simulink model "LHC_18kW_v3"  (R2015a)
settings: Solver=ode15s  StartTime=0.0  StopTime=5e6  MaxStep=1e2  RelTol=1e-3
libraries: simCryogenics_lib x134, nesl_utility x90
(part 2 of 2)

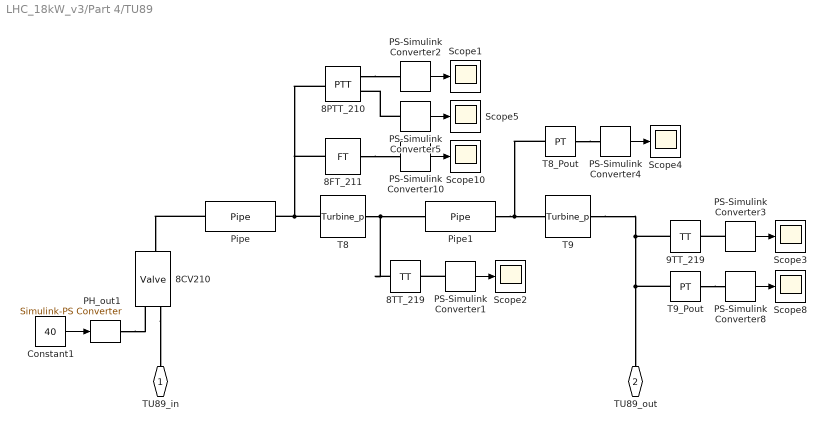
== system LHC_18kW_v3/Part 4/TU89 ==
  8CV210 : simCryogenics_lib/Elements/Valve  CVmax=37  ControlInputMin=0  ControlInputMax=100  Xt=0.65  Rv=50  lin_v=0  lim_v=0  K=2.4e-5 m^1.50000*kg^0.50000/s/bar^0.50000  Cmd_specify=off  Cmd_priority=High  Cmd=0  gamma_specify=off  gamma_priority=High  gamma=0  rho_specify=off  rho_priority=High  rho=0 kg/m^3  Xc_specify=off  Xc_priority=High  Xc=0  X_specify=off  X_priority=High  X=0  Y_specify=off  Y_priority=High  Y=0  CV_specify=off  CV_priority=High  CV=0
  8FT_211 : simCryogenics_lib/Sensors/FT
  8PTT_210 : simCryogenics_lib/Sensors/PTT
  8TT_219 : simCryogenics_lib/Sensors/TT
  9TT_219 : simCryogenics_lib/Sensors/TT
  Constant1 : Constant  Value=40
  PH_out1 : nesl_utility/Simulink-PS Converter  PhysicalDomain=network_engine_domain  SubClassName=ps_input  LeftPortType=input  RightPortType=output  PseudoPeriodic=off  Frequencies=[]  NoiseDistribution=none  NoiseParameters=[]  Unit=bar  AffineConversion=off  InputFiltering=off  SimscapeFilterOrder=1  InputFilterTimeConstant=0.001  UdotUserProvided=1
  PS-Simulink Converter{1..5,8,10} (7 alike) : nesl_utility/PS-Simulink Converter  PhysicalDomain=network_engine_domain  SubClassName=ps_output  LeftPortType=input  RightPortType=output  PseudoPeriodic=off  Frequencies=[]  Unit=1  AffineConversion=off
  Pipe : simCryogenics_lib/Elements/Pipe  Vol=1 m^3  Ideal=0  P0=13 bar  T0=19.6 K
  Pipe1 : simCryogenics_lib/Elements/Pipe  Vol=1 m^3  Ideal=0  P0=4.6 bar  T0=14.4 K
  Scope{1..5,8,10} (7 alike) : Scope
      Scope1 settings: TimeRange=10000  YMin=13.3947  YMax=13.3947  SaveName=ScopeData32
      Scope10 settings: TimeRange=10000  SaveName=ScopeData34
      Scope2 settings: TimeRange=10000  YMin=100  YMax=180  SaveName=ScopeData63
      Scope3 settings: TimeRange=10000  YMin=100  YMax=180  SaveName=ScopeData45
      Scope4 settings: TimeRange=10000  SaveName=ScopeData64
      Scope5 settings: TimeRange=10000  YMin=24.6307  YMax=24.6308  SaveName=ScopeData33
      Scope8 settings: TimeRange=10000  SaveName=ScopeData46
  T8 : simCryogenics_lib/Elements/Turbine_p  A=5.8341e-05 m^2  D=0.020 m  Mass=10 kg  cst_eff=0  eta0=0.76  Tin0=19.6 K  Pin0=12.8 bar  Pout0=3.76 bar  N0=2200 1/s  Q0=0 W  v0=0  I=0 kg*m^2  gamma_specify=off  gamma_priority=High  gamma=0  C_specify=off  C_priority=High  C=0  Z_specify=off  Z_priority=High  Z=0  Cp_specify=off  Cp_priority=High  Cp=0 kJ/kg/K  Sin_specify=off  Sin_priority=High  Sin=0 kJ/kg  T_specify=off  T_priority=High  T=0 K  HoutIs_specify=off  HoutIs_priority=High  HoutIs=0 kJ/kg  u1_specify=off  u1_priority=High  u1=0 m/s  c1_specify=off  c1_priority=High  c1=0 m/s  v_specify=off  v_priority=High  v=0  eta_specify=off  eta_priority=High  eta=0  eta_var_specify=off  eta_var_priority=High  eta_var=0  N_specify=off  N_priority=High  N=0 rad/s  Q_specify=off  Q_priority=High  Q=0 W
  T8_Pout : simCryogenics_lib/Sensors/PT
  T9 : simCryogenics_lib/Elements/Turbine_p  A=1.3750e-04 m^2  D=0.0283 m  Mass=10 kg  cst_eff=0  eta0=0.79  Tin0=14.4 K  Pin0=4.6 bar  Pout0=1.21 bar  N0=1367 1/s  Q0=0 W  v0=0  I=0 kg*m^2  gamma_specify=off  gamma_priority=High  gamma=0  C_specify=off  C_priority=High  C=0  Z_specify=off  Z_priority=High  Z=0  Cp_specify=off  Cp_priority=High  Cp=0 kJ/kg/K  Sin_specify=off  Sin_priority=High  Sin=0 kJ/kg  T_specify=off  T_priority=High  T=0 K  HoutIs_specify=off  HoutIs_priority=High  HoutIs=0 kJ/kg  u1_specify=off  u1_priority=High  u1=0 m/s  c1_specify=off  c1_priority=High  c1=0 m/s  v_specify=off  v_priority=High  v=0  eta_specify=off  eta_priority=High  eta=0  eta_var_specify=off  eta_var_priority=High  eta_var=0  N_specify=off  N_priority=High  N=0 rad/s  Q_specify=off  Q_priority=High  Q=0 W
  T9_Pout : simCryogenics_lib/Sensors/PT
  TU89_in : PMIOPort  Port=1  Side=Left
  TU89_out : PMIOPort  Port=2  Side=Right
  wires:
  Constant1/1 -> PH_out1/1
  PS-Simulink Converter5/1 -> Scope5/1
  PS-Simulink Converter10/1 -> Scope10/1
  PS-Simulink Converter2/1 -> Scope1/1
  PS-Simulink Converter3/1 -> Scope3/1
  PS-Simulink Converter8/1 -> Scope8/1
  PS-Simulink Converter1/1 -> Scope2/1
  PS-Simulink Converter4/1 -> Scope4/1
  connections:
  PH_out1/RConn1 -- 8CV210/LConn1
  8CV210/LConn2 -- TU89_in/RConn1
  T8/LConn1 -- 8FT_211/LConn1 -- 8PTT_210/LConn1 -- Pipe/RConn1
  Pipe/LConn1 -- 8CV210/RConn1
  9TT_219/LConn1 -- T9/RConn1 -- T9_Pout/LConn1 -- TU89_out/RConn1
  8PTT_210/RConn1 -- PS-Simulink Converter2/LConn1
  PS-Simulink Converter5/LConn1 -- 8PTT_210/RConn2
  8FT_211/RConn1 -- PS-Simulink Converter10/LConn1
  T9_Pout/RConn1 -- PS-Simulink Converter8/LConn1
  PS-Simulink Converter3/LConn1 -- 9TT_219/RConn1
  T8/RConn1 -- 8TT_219/LConn1 -- Pipe1/LConn1
  Pipe1/RConn1 -- T8_Pout/LConn1 -- T9/LConn1
  PS-Simulink Converter1/LConn1 -- 8TT_219/RConn1
  T8_Pout/RConn1 -- PS-Simulink Converter4/LConn1

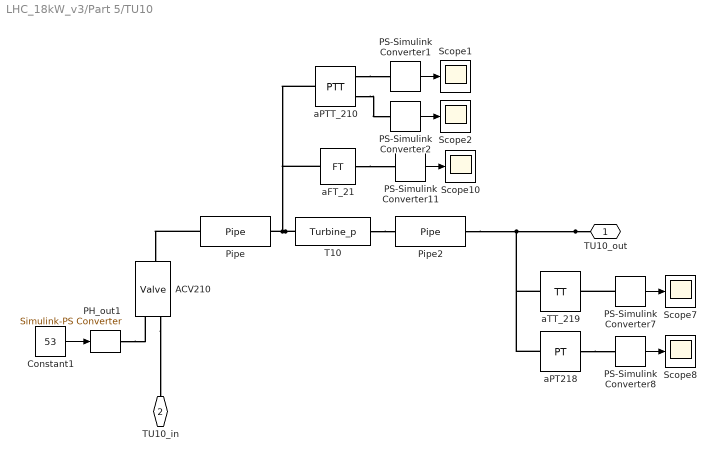
== system LHC_18kW_v3/Part 5/TU10 ==
  ACV210 : simCryogenics_lib/Elements/Valve  CVmax=11  ControlInputMin=0  ControlInputMax=100  Xt=0.65  Rv=50  lin_v=0  lim_v=0  K=2.4e-5 m^1.50000*kg^0.50000/s/bar^0.50000  Cmd_specify=off  Cmd_priority=High  Cmd=0  gamma_specify=off  gamma_priority=High  gamma=0  rho_specify=off  rho_priority=High  rho=0 kg/m^3  Xc_specify=off  Xc_priority=High  Xc=0  X_specify=off  X_priority=High  X=0  Y_specify=off  Y_priority=High  Y=0  CV_specify=off  CV_priority=High  CV=0
  Constant1 : Constant  Value=53
  PH_out1 : nesl_utility/Simulink-PS Converter  PhysicalDomain=network_engine_domain  SubClassName=ps_input  LeftPortType=input  RightPortType=output  PseudoPeriodic=off  Frequencies=[]  NoiseDistribution=none  NoiseParameters=[]  Unit=bar  AffineConversion=off  InputFiltering=off  SimscapeFilterOrder=1  InputFilterTimeConstant=0.001  UdotUserProvided=1
  PS-Simulink Converter{1..2,7..8,11} (5 alike) : nesl_utility/PS-Simulink Converter  PhysicalDomain=network_engine_domain  SubClassName=ps_output  LeftPortType=input  RightPortType=output  PseudoPeriodic=off  Frequencies=[]  Unit=1  AffineConversion=off
  Pipe : simCryogenics_lib/Elements/Pipe  Vol=1 m^3  Ideal=0  P0=13 bar  T0=8.1 K
  Pipe2 : simCryogenics_lib/Elements/Pipe  Vol=1 m^3  Ideal=0  P0=1.5 bar  T0=4.6 K
  Scope{1..2,7..8,10} (5 alike) : Scope
      Scope1 settings: TimeRange=10000  YMin=12.8609  YMax=12.8609  SaveName=ScopeData5
      Scope10 settings: TimeRange=10000  YMin=0.302619  YMax=0.302619  SaveName=ScopeData52
      Scope2 settings: TimeRange=10000  YMin=5.44996  YMax=5.44996  SaveName=ScopeData13
      Scope7 settings: TimeRange=10000  SaveName=ScopeData53
      Scope8 settings: TimeRange=10000  SaveName=ScopeData54
  T10 : simCryogenics_lib/Elements/Turbine_p  A=3.1203e-05 m^2  D=0.0137 m  Mass=1.8 kg  cst_eff=1  eta0=0.72  Tin0=8.1 K  Pin0=12.8 bar  Pout0=2.98 bar  N0=1690 1/s  Q0=0 W  v0=0  I=0 kg*m^2  gamma_specify=off  gamma_priority=High  gamma=0  C_specify=off  C_priority=High  C=0  Z_specify=off  Z_priority=High  Z=0  Cp_specify=off  Cp_priority=High  Cp=0 kJ/kg/K  Sin_specify=off  Sin_priority=High  Sin=0 kJ/kg  T_specify=off  T_priority=High  T=0 K  HoutIs_specify=off  HoutIs_priority=High  HoutIs=0 kJ/kg  u1_specify=off  u1_priority=High  u1=0 m/s  c1_specify=off  c1_priority=High  c1=0 m/s  v_specify=off  v_priority=High  v=0  eta_specify=off  eta_priority=High  eta=0  eta_var_specify=off  eta_var_priority=High  eta_var=0  N_specify=off  N_priority=High  N=0 rad/s  Q_specify=off  Q_priority=High  Q=0 W
  aFT_21 : simCryogenics_lib/Sensors/FT
  aPT218 : simCryogenics_lib/Sensors/PT
  aPTT_210 : simCryogenics_lib/Sensors/PTT
  aTT_219 : simCryogenics_lib/Sensors/TT
  TU10_out : PMIOPort  Port=1  Side=Right
  TU10_in : PMIOPort  Port=2  Side=Left
  wires:
  PS-Simulink Converter8/1 -> Scope8/1
  PS-Simulink Converter7/1 -> Scope7/1
  PS-Simulink Converter11/1 -> Scope10/1
  PS-Simulink Converter1/1 -> Scope1/1
  PS-Simulink Converter2/1 -> Scope2/1
  Constant1/1 -> PH_out1/1
  connections:
  PS-Simulink Converter7/LConn1 -- aTT_219/RConn1
  aPT218/RConn1 -- PS-Simulink Converter8/LConn1
  aFT_21/RConn1 -- PS-Simulink Converter11/LConn1
  aPTT_210/RConn1 -- PS-Simulink Converter1/LConn1
  aPTT_210/RConn2 -- PS-Simulink Converter2/LConn1
  PH_out1/RConn1 -- ACV210/LConn1
  Pipe/LConn1 -- ACV210/RConn1
  T10/RConn1 -- Pipe2/LConn1
  TU10_out/RConn1 -- aTT_219/LConn1 -- aPT218/LConn1 -- Pipe2/RConn1
  ACV210/LConn2 -- TU10_in/RConn1
  Pipe/RConn1 -- aPTT_210/LConn1 -- aFT_21/LConn1 -- T10/LConn1

== system LHC_18kW_v3/Part 5/gain ==
  Bias2 : Bias  Bias=55
  Bias3 : Bias  Bias=-2.7
  Gain1 : Gain  Gain=100
  PH_out4 : nesl_utility/Simulink-PS Converter  PhysicalDomain=network_engine_domain  SubClassName=ps_input  LeftPortType=input  RightPortType=output  PseudoPeriodic=off  Frequencies=[]  NoiseDistribution=none  NoiseParameters=[]  Unit=bar  AffineConversion=off  InputFiltering=off  SimscapeFilterOrder=1  InputFilterTimeConstant=0.001  UdotUserProvided=1
  PS-Simulink Converter13 : nesl_utility/PS-Simulink Converter  PhysicalDomain=network_engine_domain  SubClassName=ps_output  LeftPortType=input  RightPortType=output  PseudoPeriodic=off  Frequencies=[]  Unit=1  AffineConversion=off
  Scope11 : Scope
      settings: TimeRange=10000  YMin=2.66  YMax=2.76  SaveName=ScopeData69
  T6_Pout : simCryogenics_lib/Sensors/PT
  Conn1 : PMIOPort  Port=1  Side=Right
  Conn2 : PMIOPort  Port=2  Side=Left
  wires:
  Bias2/1 -> PH_out4/1
  PS-Simulink Converter13/1 -> Bias3/1, Scope11/1
  Bias3/1 -> Gain1/1
  Gain1/1 -> Bias2/1
  connections:
  PH_out4/RConn1 -- Conn1/RConn1
  T6_Pout/LConn1 -- Conn2/RConn1
  T6_Pout/RConn1 -- PS-Simulink Converter13/LConn1
